simulink model "rtwdemo_other2"  (Simulink 7.1)
settings: Solver=FixedStepDiscrete  StartTime=0.0  StopTime=10.0  RelTol=1e-3
settings Model: Creator=ajayaram  LastModifiedBy=ajayaram
settings OptimizationCC: InlineParams=on  OptimizeModelRefInitCode=on  LifeSpan=1
settings DebuggingCC: SaveWithParameterizedLinksMsg=none
settings RTWCC: SystemTargetFile=ert.tlc  GenCodeOnly=on  GenerateMakefile=off  TemplateMakefile=ert_default_tmf  Description=Real-Time Workshop Embedded Coder (no auto configuration)  GenerateReport=on  ProcessScript=ert_make_rtw_hook  IncludeHyperlinkInReport=on  LaunchReport=on
settings CodeAppCC: IgnoreCustomStorageClasses=off
settings ERTTargetCC: TargetFcnLib=ansi_tfl_tmw.mat  GenerateSampleERTMain=on  InlinedParameterPlacement=NonHierarchical  ERTCustomFileTemplate=example_file_process.tlc

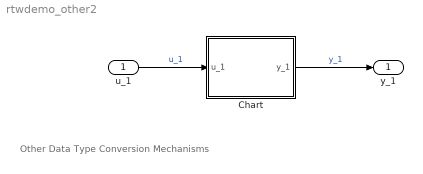
== system rtwdemo_other2 ==
  note: Other Data Type Conversion Mechanisms
  u_1 : Inport  DataType=int16  OutDataType=sfix(16)  OutScaling=2^0  OutDataTypeStr=int16
  Chart : Stateflow chart
  y_1 : Outport  OutDataType=sfix(16)  OutScaling=2^0
  wires:
  u_1/1 -> Chart/1(u_1)  "u_1"
  Chart/1(y_1) -> y_1/1  "y_1"

== stateflow chart Chart ==
  (default) -> (junction 3)
  (junction 3) -> (junction 4) : {
      | y_1 = 2* u_1;
      | }
  data: y_1 output double; u_1 input int16
